simulink model "Part_4_Simulink_Cycle_Communication_Detailled_Blocks"  (R2016a)
settings: Solver=VariableStepAuto  StartTime=0.0  StopTime=12  RelTol=1e-3
values from neighbouring files (symbols this model uses):
  Alpha = 1    [Parameters_And_Plot.m]    (also in Part5_Specified_Destinations.m)
  K15 = K(1,5)    [Parameters_And_Plot.m]    (also in Part5_Specified_Destinations.m)
  K21 = K(2,1)    [Parameters_And_Plot.m]    (also in Part5_Specified_Destinations.m)
  K32 = K(3,2)    [Parameters_And_Plot.m]    (also in Part5_Specified_Destinations.m)
  K43 = K(4,3)    [Parameters_And_Plot.m]    (also in Part5_Specified_Destinations.m)
  K54 = K(5,4)    [Parameters_And_Plot.m]    (also in Part5_Specified_Destinations.m)
  L = 1    [Parameters_And_Plot.m]    (also in Part5_Specified_Destinations.m)
  x1_0 = r1_0(1)    [Parameters_And_Plot.m]    (also in Part5_Specified_Destinations.m)
  x1d = r1d(1)    [Parameters_And_Plot.m]    (also in Part5_Specified_Destinations.m)
  x2_0 = r2_0(1)    [Parameters_And_Plot.m]    (also in Part5_Specified_Destinations.m)
  x2d = r2d(1)    [Parameters_And_Plot.m]    (also in Part5_Specified_Destinations.m)
  x3_0 = r3_0(1)    [Parameters_And_Plot.m]    (also in Part5_Specified_Destinations.m)
  x3d = r3d(1)    [Parameters_And_Plot.m]    (also in Part5_Specified_Destinations.m)
  x4_0 = r4_0(1)    [Parameters_And_Plot.m]    (also in Part5_Specified_Destinations.m)
  x4d = r4d(1)    [Parameters_And_Plot.m]    (also in Part5_Specified_Destinations.m)
  x5_0 = r5_0(1)    [Parameters_And_Plot.m]    (also in Part5_Specified_Destinations.m)
  x5d = r5d(1)    [Parameters_And_Plot.m]    (also in Part5_Specified_Destinations.m)
  y1_0 = r1_0(2)    [Parameters_And_Plot.m]    (also in Part5_Specified_Destinations.m)
  y1d = r1d(2)    [Parameters_And_Plot.m]    (also in Part5_Specified_Destinations.m)
  y2_0 = r2_0(2)    [Parameters_And_Plot.m]    (also in Part5_Specified_Destinations.m)
  y2d = r2d(2)    [Parameters_And_Plot.m]    (also in Part5_Specified_Destinations.m)
  y3_0 = r3_0(2)    [Parameters_And_Plot.m]    (also in Part5_Specified_Destinations.m)
  y3d = r3d(2)    [Parameters_And_Plot.m]    (also in Part5_Specified_Destinations.m)
  y4_0 = r4_0(2)    [Parameters_And_Plot.m]    (also in Part5_Specified_Destinations.m)
  y4d = r4d(2)    [Parameters_And_Plot.m]    (also in Part5_Specified_Destinations.m)
  y5_0 = r5_0(2)    [Parameters_And_Plot.m]    (also in Part5_Specified_Destinations.m)
  y5d = r5d(2)    [Parameters_And_Plot.m]    (also in Part5_Specified_Destinations.m)
settings Model: Creator=Mohammad Hammoud  LastModifiedBy=Mohammad Hammoud

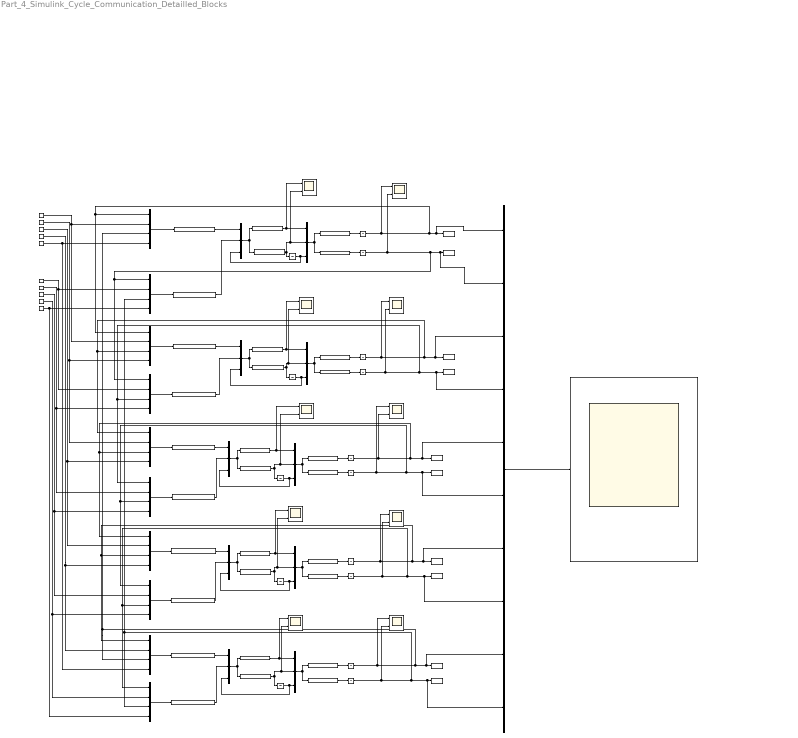
== system Part_4_Simulink_Cycle_Communication_Detailled_Blocks ==
  note: < Robot 2
  note: ^
      | Robot 1
      | v
  note: Yi desired
  note: Xi desired
  note: Consensus-based Conrol Law (New)
  note: In these Scopes we can see the Graphs of Linear
      | displacements Xi and Yi for each Robot alone
  note: In these Scopes we can see the Graphs of Linear Velocity
      | Vi and Angular Velocity Wi for each Robot alone
  note: Scope to show all Linear Displacements
      | Xi and Yi of All Robots, function of Time
  note: We chose the Cyclic Graph of Communication between Robots
      | ---> Each robot can take information from the previous one, and give information to the next robot (this forms a one-way cycle)
  note: Part 4: " P ropose another simplified graph with less connections, which
      | responds to the problem; then adapt the proposed controller "
  note: x1
  note: < Robot 3
  note: < Robot 4
  note: < Robot 5
  Constant10 : Constant  Value=y3d
  Constant11 : Constant  Value=y4d
  Constant12 : Constant  Value=y5d
  Constant3 : Constant  Value=x1d
  Constant4 : Constant  Value=x2d
  Constant5 : Constant  Value=x3d
  Constant6 : Constant  Value=x4d
  Constant7 : Constant  Value=x5d
  Constant8 : Constant  Value=y1d
  Constant9 : Constant  Value=y2d
  Integrator{,1,4,6,10} (5 alike) : Integrator
  "Integrator1 " : Integrator  InitialCondition=x1_0
  "Integrator10 " : Integrator  InitialCondition=y4_0
  "Integrator11 " : Integrator  InitialCondition=x5_0
  "Integrator12 " : Integrator  InitialCondition=y5_0
  Integrator2 : Integrator  InitialCondition=y1_0
  Integrator3 : Integrator  InitialCondition=y2_0
  "Integrator4 " : Integrator  InitialCondition=x2_0
  "Integrator5 " : Integrator  InitialCondition=x3_0
  "Integrator8 " : Integrator  InitialCondition=y3_0
  "Integrator9 " : Integrator  InitialCondition=x4_0
  Mux{,1..4,7,10,13,16,20} (10 alike) : Mux
  Mux{5..6,8..9,11..12,14..15,21..22} (10 alike) : Mux  Inputs=3
  Mux17 : Mux  Inputs=10
  Scope : Scope
  Scope{1..10} (10 alike) : Scope  NumInputPorts=2
  To Workspace1 : ToWorkspace  VariableName=xh1  SampleTime=-1
  To Workspace11 : ToWorkspace  VariableName=xh3  SampleTime=-1
  To Workspace12 : ToWorkspace  VariableName=yh3  SampleTime=-1
  To Workspace2 : ToWorkspace  VariableName=yh1  SampleTime=-1
  To Workspace3 : ToWorkspace  VariableName=xh2  SampleTime=-1
  To Workspace4 : ToWorkspace  VariableName=yh2  SampleTime=-1
  To Workspace5 : ToWorkspace  VariableName=xh5  SampleTime=-1
  To Workspace6 : ToWorkspace  VariableName=xh4  SampleTime=-1
  To Workspace7 : ToWorkspace  VariableName=yh4  SampleTime=-1
  To Workspace8 : ToWorkspace  VariableName=yh5  SampleTime=-1
  Ux1 : Fcn  Expr=-Alpha*(u(1)-u(2)) - K15 * ((u(1) - u(2)) - (u(3) - u(4)))
  Ux2 : Fcn  Expr=-Alpha * (u(3) - u(4)) - K21 * ((u(3) - u(4)) - (u(1) - u(2)))
  Ux3 : Fcn  Expr=-Alpha * (u(3) - u(4)) - K32 * ((u(3) - u(4)) - (u(1) - u(2)))
  Ux4 : Fcn  Expr=-Alpha * (u(3) - u(4)) - K43 * ((u(3) - u(4)) - (u(1) - u(2)))
  Ux5 : Fcn  Expr=-Alpha * (u(3) - u(4)) - K54 * ((u(3) - u(4)) - (u(1) - u(2)))
  Uy1 : Fcn  Expr=-Alpha*(u(1)-u(2)) - K15 * ((u(1) - u(2)) - (u(3) - u(4)))
  Uy2 : Fcn  Expr=-Alpha * (u(3) - u(4)) - K21 * ((u(3) - u(4)) - (u(1) - u(2)))
  Uy3 : Fcn  Expr=-Alpha * (u(3) - u(4)) - K32 * ((u(3) - u(4)) - (u(1) - u(2)))
  Uy4 : Fcn  Expr=-Alpha * (u(3) - u(4)) - K43 * ((u(3) - u(4)) - (u(1) - u(2)))
  Uy5 : Fcn  Expr=-Alpha * (u(3) - u(4)) - K54 * ((u(3) - u(4)) - (u(1) - u(2)))
  V{1..5} (5 alike) : Fcn  Expr=u(1)*cos(u(3)) + u(2)*sin(u(3))
  W{1..5} (5 alike) : Fcn  Expr=-(u(1)*sin(u(3)))/L + (u(2)*cos(u(3)))/L
  Xhdot {1..5} (5 alike) : Fcn  Expr=u(1)*cos(u(3)) - L*u(2)*sin(u(3))
  Yhdot {1..5} (5 alike) : Fcn  Expr=u(1)*sin(u(3)) + L*u(2)*cos(u(3))
  wires:
  Constant3/1 -> Mux20/2, Mux/2  "x1d"
  Mux/1 -> Ux1/1
  Constant4/1 -> Mux10/2, Mux20/4  "x2d"
  Constant5/1 -> Mux3/2, Mux10/4  "x3d"
  Constant6/1 -> Mux4/2, Mux3/4  "x4d"
  Constant7/1 -> Mux4/4, Mux/4  "x5d"
  Constant8/1 -> Mux7/2, Mux1/2  "y1d"
  Mux1/1 -> Uy1/1
  Constant9/1 -> Mux2/2, Mux7/4  "y2d"
  Constant10/1 -> Mux13/2, Mux2/4  "y3d"
  Constant11/1 -> Mux16/2, Mux13/4  "y4d"
  Constant12/1 -> Mux16/4, Mux1/4  "y5d"
  Mux2/1 -> Uy3/1
  Mux4/1 -> Ux5/1
  Mux5/1 -> V1/1, W1/1
  Integrator/1 -> Mux6/3, Mux5/3  "Theta 1"
  V1/1 -> Scope1/1, Mux6/1  "V1"
  W1/1 -> Scope1/2, Mux6/2, Integrator/1  "W1"
  Mux6/1 -> Xhdot 1/1, Yhdot 1/1
  Yhdot 1/1 -> Integrator2/1
  Xhdot 1/1 -> "Integrator1 "/1
  "Integrator1 "/1 -> Scope4/1, Mux20/1, Mux/1, Mux17/1, To Workspace1/1  "x1"
  Integrator2/1 -> Scope4/2, Mux7/1, Mux1/1, Mux17/2, To Workspace2/1  "y1"
  Mux8/1 -> V2/1, W2/1
  Integrator1/1 -> Mux8/3, Mux9/3  "Theta 2"
  V2/1 -> Scope2/1, Mux9/1  "V2"
  W2/1 -> Integrator1/1, Scope2/2, Mux9/2  "W2"
  Mux9/1 -> Yhdot 2/1, Xhdot 2/1
  Yhdot 2/1 -> Integrator3/1
  Xhdot 2/1 -> "Integrator4 "/1
  "Integrator4 "/1 -> Scope3/1, Mux17/3, To Workspace3/1, Mux10/1, Mux20/3  "x2"
  Integrator3/1 -> Scope3/2, Mux17/4, To Workspace4/1, Mux2/1, Mux7/3  "y2"
  Uy3/1 -> Mux21/2  "Uy3"
  Ux1/1 -> Mux5/1  "Ux1"
  Uy1/1 -> Mux5/2  "Uy1"
  Mux20/1 -> Ux2/1
  Ux2/1 -> Mux8/1  "Ux2"
  Mux7/1 -> Uy2/1
  Uy2/1 -> Mux8/2  "Uy2"
  Mux10/1 -> Ux3/1
  Mux21/1 -> V3/1, W3/1
  Integrator10/1 -> Mux21/3, Mux22/3  "Theta 3"
  V3/1 -> Scope5/1, Mux22/1  "V3"
  W3/1 -> Integrator10/1, Scope5/2, Mux22/2  "W3"
  Mux22/1 -> Yhdot 3/1, Xhdot 3/1
  Yhdot 3/1 -> "Integrator8 "/1
  Xhdot 3/1 -> "Integrator5 "/1
  "Integrator5 "/1 -> Mux3/1, Mux10/3, Mux17/5, To Workspace11/1, Scope6/2  "x3"
  "Integrator8 "/1 -> Scope6/1, Mux17/6, To Workspace12/1, Mux13/1, Mux2/3  "y3"
  Ux3/1 -> Mux21/1  "Ux3"
  Mux3/1 -> Ux4/1
  Mux11/1 -> V4/1, W4/1
  Integrator4/1 -> Mux11/3, Mux12/3  "Theta 4"
  V4/1 -> Scope7/1, Mux12/1  "V4"
  W4/1 -> Integrator4/1, Mux12/2, Scope7/2  "W4"
  Mux12/1 -> Yhdot 4/1, Xhdot 4/1
  Yhdot 4/1 -> "Integrator10 "/1
  Xhdot 4/1 -> "Integrator9 "/1
  "Integrator9 "/1 -> Scope8/1, Mux4/1, Mux3/3, Mux17/7, To Workspace6/1  "x4"
  "Integrator10 "/1 -> Scope8/2, Mux16/1, Mux13/3, Mux17/8, To Workspace7/1  "y4"
  Ux4/1 -> Mux11/1  "Ux4"
  Mux13/1 -> Uy4/1
  Uy4/1 -> Mux11/2  "Uy4"
  Mux14/1 -> V5/1, W5/1
  Integrator6/1 -> Mux14/3, Mux15/3  "Theta 5"
  V5/1 -> Scope9/1, Mux15/1  "V5"
  W5/1 -> Integrator6/1, Mux15/2, Scope9/2  "W5"
  Mux15/1 -> Yhdot 5/1, Xhdot 5/1
  Yhdot 5/1 -> "Integrator12 "/1
  Xhdot 5/1 -> "Integrator11 "/1
  "Integrator11 "/1 -> Scope10/1, Mux4/3, Mux/3, Mux17/9, To Workspace5/1  "x5"
  "Integrator12 "/1 -> Mux16/3, Mux1/3, Mux17/10, To Workspace8/1, Scope10/2  "y5"
  Ux5/1 -> Mux14/1  "Ux5"
  Mux16/1 -> Uy5/1
  Uy5/1 -> Mux14/2  "Uy5"
  Mux17/1 -> Scope/1
